simulink library "libForecasters"  (R2015a)
settings: Solver=ode45  StartTime=0.0  StopTime=10.0  RelTol=1e-3
libraries: libForecasters x1
settings Model: Creator=jcardena  LastModifiedBy=jcardena

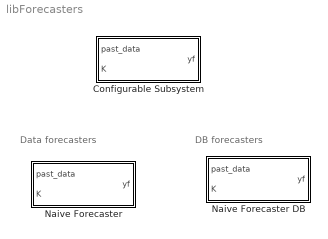
== system libForecasters ==
  note: DB forecasters
  note: Data forecasters
  Configurable Subsystem : Subsystem  BlockChoice=Naive Forecaster
      settings: TemplateBlock=self  MemberBlocks=Naive Forecaster,Naive Forecaster DB
  Naive Forecaster : Subsystem
      mask Display: image('images/forecast_icon.png')
  Naive Forecaster DB : Subsystem

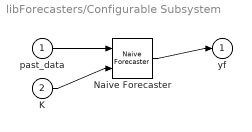
== system libForecasters/Configurable Subsystem ==
  past_data : Inport
  K : Inport  Port=2
  Naive Forecaster : libForecasters/Naive Forecaster  SystemSampleTime=-1
  yf : Outport
  wires:
  past_data/1 -> Naive Forecaster/1
  K/1 -> Naive Forecaster/2
  Naive Forecaster/1 -> yf/1

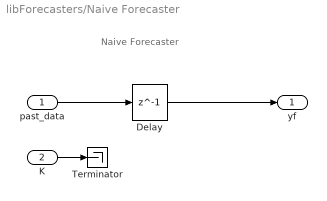
== system libForecasters/Naive Forecaster ==
  note: Naive Forecaster
  past_data : Inport
  K : Inport  Port=2
  Delay : Delay  DelayLength=1  InitialCondition=0
  Terminator : Terminator
  yf : Outport
  wires:
  past_data/1 -> Delay/1
  Delay/1 -> yf/1
  K/1 -> Terminator/1

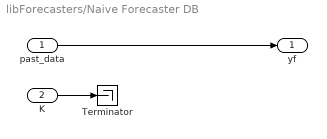
== system libForecasters/Naive Forecaster DB ==
  past_data : Inport
  K : Inport  Port=2
  Terminator : Terminator
  yf : Outport
  wires:
  past_data/1 -> yf/1
  K/1 -> Terminator/1
